simulink model "failureInputReadOctarotor"  (R2026a)
settings: Solver=ode4  FixedStep=stepSize_s
settings Model: Creator=Edison Altamirano  LastModifiedBy=Edison Altamirano

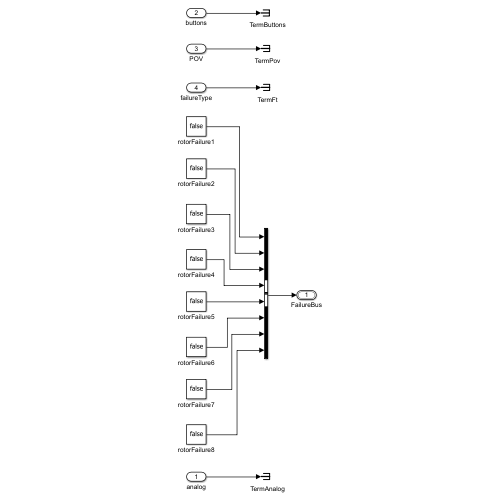
[thumbnail: Simulink's stored preview of the top-level diagram]
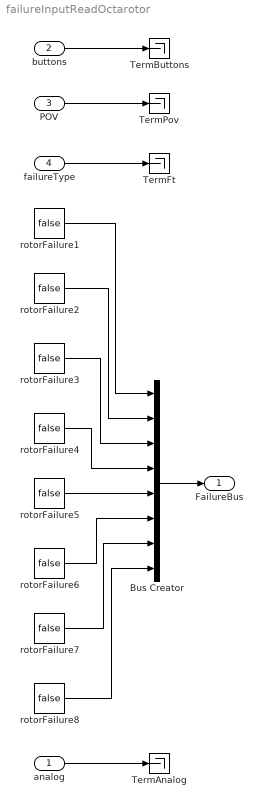
== system failureInputReadOctarotor ==
  analog : Inport  PortDimensions=6
  buttons : Inport  Port=2  OutDataTypeStr=uint32
  POV : Inport  Port=3
  failureType : Inport  Port=4  OutDataTypeStr=Enum: EnumHexFailureType
  Bus Creator : BusCreator  Inputs=8
  TermAnalog : Terminator
  TermButtons : Terminator
  TermFt : Terminator
  TermPov : Terminator
  rotorFailure{1..8} (8 alike) : Constant  Value=false
  FailureBus : Outport  OutDataTypeStr=Bus: FailureBus
  wires:
  Bus Creator/1 -> FailureBus/1
  rotorFailure8/1 -> Bus Creator/8
  rotorFailure7/1 -> Bus Creator/7
  rotorFailure6/1 -> Bus Creator/6
  rotorFailure5/1 -> Bus Creator/5
  rotorFailure4/1 -> Bus Creator/4
  rotorFailure3/1 -> Bus Creator/3
  rotorFailure2/1 -> Bus Creator/2
  rotorFailure1/1 -> Bus Creator/1
  failureType/1 -> TermFt/1
  POV/1 -> TermPov/1
  buttons/1 -> TermButtons/1
  analog/1 -> TermAnalog/1
